simulink model "Hexa_CAD_ANSFT_Sim"  (R2024b)
settings: Solver=ode4  StartTime=0.0  StopTime=8  FixedStep=0.01  RelTol=1e-3
model workspace (MAT data in the model file):
  hover_2m = [0 0 2 0 0 0 0 0 2 0 0 0 ... (36 elements, 6x6)]
  square = [0 0 2.5 0 0 0 0 0 2.5 0 0 0 ... (36 elements, 6x6)]
  tf : Simulink.Parameter (value not decoded)
  tray0 = [0 0 0 0 0 0 0.2 0.15 2 0 0 0 ... (36 elements, 6x6)]
  tray1 = [0 0 0 0 0 0 0 0 5 0 0 0 ... (36 elements, 6x6)]
  tray2 = [0 0 0 0 0 0 2 0 5 0 0 0 ... (36 elements, 6x6)]
  tray3 = [0 0 0 0 0 0 2 0 5 0 0 0 ... (36 elements, 6x6)]
  tray4 = [0 0 0 0 0 0 2 0 5 0.15 0 0 ... (36 elements, 6x6)]
  tray5 = [0 0 0 0 0 0 0 0 5 0.15 0 0 ... (36 elements, 6x6)]
  tray_yaw = [0 0 0 0 0 0 0 0 5 0 0 0 ... (36 elements, 6x6)]
undefined symbols (not defined in the file or in its folder): F, Light, MIL, smiData, X, Y, Z
libraries: sm_lib x238, nesl_utility x29, dspobslib x7, simulink x3, sharedtransform x2, robotcorelib x1, aerolibwind2 x1
(part 2 of 6)

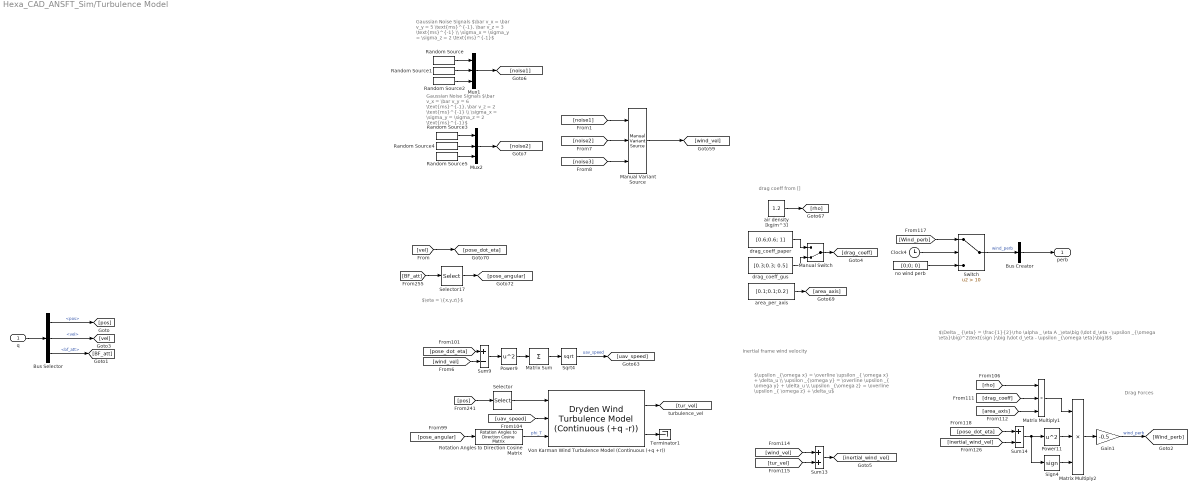
== system Hexa_CAD_ANSFT_Sim/Turbulence Model ==
  note: $\Delta _ {\eta} = \frac{1}{2}\rho \alpha _ \eta A _\eta\big (\dot d_\eta - \upsilon _{\omega \eta}\big)^2\text{sign }\big (\dot d_\eta - \upsilon _{\omega \eta}\big)$$
  note: $\upsilon _{\omega x} = \overline \upsilon _{ \omega x} + \delta_u \\ \upsilon _{\omega y} = \overline \upsilon _{ \omega y} + \delta_u \\ \upsilon _{\omega z} = \overline \upsilon _{ \omega z} + \delta_u$
  note: drag coeff from []
  note: Drag Forces
  note: Inertial frame wind velocity
  note: $\eta = \{x,y,z\}$
  note: Gaussian Noise Signals
      | $\bar v_x = \bar v_y = 6 \text{ms}^{-1}, \bar v_z = 2 \text{ms}^{-1} \\ \sigma_x = \sigma_y = \sigma_z = 2 \text{ms}^{-1}$
  note: Gaussian Noise Signals
      | $\bar v_x = \bar v_y = 5 \text{ms}^{-1}, \bar v_z = 3 \text{ms}^{-1} \\ \sigma_x = \sigma_y = \sigma_z = 2 \text{ms}^{-1}$
  q : Inport
  Bus Creator : BusCreator  Inputs=1
  Bus Selector : BusSelector  OutputSignals=pos,vel,bf_att
  Clock4 : Clock
  Gain1 : Gain  Gain=-0.5
  Manual Variant Source : simulink/Signal Routing/Manual Variant Source  NumChoices=3  LabelModeActiveChoice=V_1
  Manual Switch : ManualSwitch  CurrentSetting=0
  Matrix Sum : Sum  Inputs=+
  Matrix Multiply1 : Product  Inputs=3
  Matrix Multiply2 : Product  Inputs=3
  Mux1 : Mux  Inputs=3
  Mux2 : Mux  Inputs=3
  Power11 : Math  Operator=square
  Power9 : Math  Operator=square
  Random Source : dspobslib/Random Source  SrcType=Gaussian  NormMethod=Ziggurat  CltLength=12  MinVal=0  MaxVal=1  MeanVal=5  VarVal=2  RepMode=Not repeatable  rawSeed=1  IsInherit=off  SampMode=Discrete  SampTime=1  SampFrame=1  DataType=Double  OutComplex=Real  OutputFrames=off
  Random Source1 : dspobslib/Random Source  SrcType=Gaussian  NormMethod=Ziggurat  CltLength=12  MinVal=0  MaxVal=1  MeanVal=5  VarVal=2  RepMode=Not repeatable  rawSeed=1  IsInherit=off  SampMode=Discrete  SampTime=1  SampFrame=1  DataType=Double  OutComplex=Real  OutputFrames=off
  Random Source2 : dspobslib/Random Source  SrcType=Gaussian  NormMethod=Ziggurat  CltLength=12  MinVal=0  MaxVal=1  MeanVal=3  VarVal=2  RepMode=Not repeatable  rawSeed=1  IsInherit=off  SampMode=Discrete  SampTime=1  SampFrame=1  DataType=Double  OutComplex=Real  OutputFrames=off
  Random Source3 : dspobslib/Random Source  SrcType=Gaussian  NormMethod=Ziggurat  CltLength=12  MinVal=0  MaxVal=1  MeanVal=6  VarVal=2  RepMode=Not repeatable  rawSeed=1  IsInherit=off  SampMode=Discrete  SampTime=1  SampFrame=1  DataType=Double  OutComplex=Real  OutputFrames=off
  Random Source4 : dspobslib/Random Source  SrcType=Gaussian  NormMethod=Ziggurat  CltLength=12  MinVal=0  MaxVal=1  MeanVal=6  VarVal=2  RepMode=Not repeatable  rawSeed=1  IsInherit=off  SampMode=Discrete  SampTime=1  SampFrame=1  DataType=Double  OutComplex=Real  OutputFrames=off
  Random Source5 : dspobslib/Random Source  SrcType=Gaussian  NormMethod=Ziggurat  CltLength=12  MinVal=0  MaxVal=1  MeanVal=2  VarVal=2  RepMode=Not repeatable  rawSeed=1  IsInherit=off  SampMode=Discrete  SampTime=1  SampFrame=1  DataType=Double  OutComplex=Real  OutputFrames=off
  Rotation Angles to Direction Cosine Matrix : sharedtransform/Rotation Angles to Direction Cosine Matrix  rotationOrder=XYZ  aMode=aMode
  Selector : Selector  InputPortWidth=3  IndexOptions=Index vector (dialog)  Indices=[3]  OutputSizes=1
  Selector17 : Selector  InputPortWidth=3  IndexOptions=Index vector (dialog)  Indices=[3 2 1]  OutputSizes=1
  Sign4 : Signum
  Sqrt4 : Sqrt
  Sum13 : Sum
  Sum14 : Sum  Inputs=+-
  Sum9 : Sum  Inputs=+-
  Switch : Switch  Criteria=u2 > Threshold  Threshold=10  SaturateOnIntegerOverflow=off  InputSameDT=off
  Terminator1 : Terminator
  Von Karman Wind Turbulence Model (Continuous (+q +r)) : aerolibwind2/Dryden Wind Turbulence Model  (Continuous (+q -r))  units=Metric (MKS)  spec=MIL-F-8785C  model=Continuous Von Karman (+q -r)  W20=15  Wdeg=0  TurbProb=10^-2 - Light  L_high=762  Wingspan=10  ts=0.1  Seed=[23341 23342 23343 23344]  T_on=on
      settings: LibrarySourceBlock=|
      | aerolibwind2/Von Karman Wind Turbulence Model
      | (Continuous (+q +r))
  air density [kg/m^3] : Constant  Value=1.2
  area_per_axis : Constant  Value=[0.1;0.1;0.2]
  drag_coeff_gus : Constant  Value=[0.3;0.3; 0.5]
  drag_coeff_paper : Constant  Value=[0.6;0.6; 1]
  no wind perb : Constant  Value=[0;0; 0]
  perb : Outport
  wires:
  [rho] -> Matrix Multiply1/1
  [drag_coeff] -> Matrix Multiply1/2
  Von Karman Wind Turbulence Model (Continuous (+q +r))/2 -> Terminator1/1
  area_per_axis/1 -> [area_axis]
  [pose_dot_eta] -> Sum14/1
  Von Karman Wind Turbulence Model (Continuous (+q +r))/1 -> [tur_vel]
  [wind_vel] -> Sum9/2
  Selector17/1 -> [pose_angular]
  Matrix Multiply1/1 -> Matrix Multiply2/1
  Sign4/1 -> Matrix Multiply2/3
  [uav_speed] -> Von Karman Wind Turbulence Model (Continuous (+q +r))/2
  Power9/1 -> Matrix Sum/1
  Sqrt4/1 -> [uav_speed]  "uav_speed"
  Gain1/1 -> [Wind_perb]  "wind_perb"
  Sum9/1 -> Power9/1
  air density [kg/m^3]/1 -> [rho]
  Clock4/1 -> Switch/2
  [pose_dot_eta] -> Sum9/1
  Rotation Angles to Direction Cosine Matrix/1 -> Von Karman Wind Turbulence Model (Continuous (+q +r))/3  "phi_T"
  [tur_vel] -> Sum13/2
  Sum14/1 -> Sign4/1, Power11/1
  no wind perb/1 -> Switch/3
  drag_coeff_gus/1 -> Manual Switch/2
  Switch/1 -> Bus Creator/1  "wind_perb"
  [area_axis] -> Matrix Multiply1/3
  Manual Switch/1 -> [drag_coeff]
  Selector/1 -> Von Karman Wind Turbulence Model (Continuous (+q +r))/1
  [pose_angular] -> Rotation Angles to Direction Cosine Matrix/1
  [inertial_wind_vel] -> Sum14/2
  Matrix Multiply2/1 -> Gain1/1
  drag_coeff_paper/1 -> Manual Switch/1
  Power11/1 -> Matrix Multiply2/2
  Matrix Sum/1 -> Sqrt4/1
  Sum13/1 -> [inertial_wind_vel]
  [Wind_perb] -> Switch/1
  [wind_vel] -> Sum13/1
  Bus Creator/1 -> perb/1
  [BF_att] -> Selector17/1
  [pos] -> Selector/1
  q/1 -> Bus Selector/1
  Bus Selector/1 -> [pos]  "<pos>"
  Bus Selector/3 -> [BF_att]  "<bf_att>"
  Bus Selector/2 -> [vel]  "<vel>"
  [vel] -> [pose_dot_eta]
  Mux2/1 -> [noise2]
  Random Source5/1 -> Mux2/3
  Random Source/1 -> Mux1/1
  Mux1/1 -> [noise1]
  Random Source2/1 -> Mux1/3
  Random Source4/1 -> Mux2/2
  Random Source3/1 -> Mux2/1
  [noise2] -> Manual Variant Source/2
  Manual Variant Source/1 -> [wind_vel]
  Random Source1/1 -> Mux1/2
  [noise1] -> Manual Variant Source/1
  [noise3] -> Manual Variant Source/3

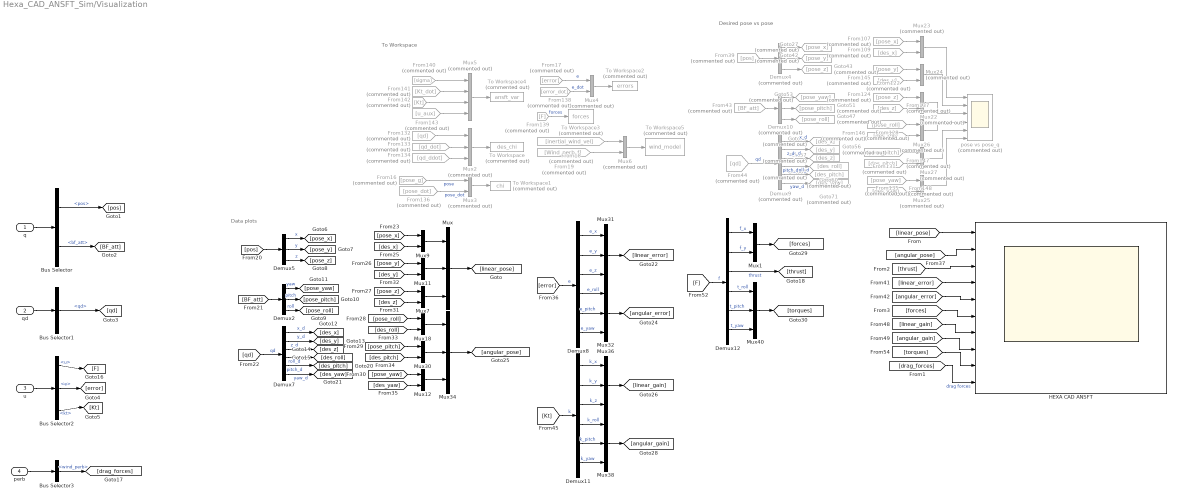
== system Hexa_CAD_ANSFT_Sim/Visualization ==
  note: Desired pose vs pose
  note: Data plots
  note: To Workspace
  q : Inport
  qd : Inport  Port=2
  u : Inport  Port=3
  perb : Inport  Port=4
  Bus Selector : BusSelector  OutputSignals=pos,bf_att
  Bus Selector1 : BusSelector  OutputSignals=qd
  Bus Selector2 : BusSelector  OutputSignals=u,e,kt
  Bus Selector3 : BusSelector  OutputSignals=wind_perb
  Demux10 : Demux  Commented=on  Outputs=3
  Demux{7..8,11..12} (4 alike) : Demux  Outputs=6
  Demux2 : Demux  Outputs=3
  Demux4 : Demux  Commented=on  Outputs=3
  Demux5 : Demux  Outputs=3
  Demux9 : Demux  Commented=on  Outputs=6
  From107 : From  Commented=on  GotoTag=pose_x
  From109 : From  Commented=on  GotoTag=des_x
  From122 : From  Commented=on  GotoTag=pose_y
  From124 : From  Commented=on  GotoTag=pose_z
  From128 : From  Commented=on  GotoTag=pose_roll
  From131 : From  Commented=on  GotoTag=pose_pitch
  From132 : From  Commented=on  GotoTag=qd
  From133 : From  Commented=on  GotoTag=qd_dot
  From134 : From  Commented=on  GotoTag=qd_ddot
  From135 : From  Commented=on  GotoTag=pose_yaw
  From136 : From  Commented=on  GotoTag=pose_dot
  From137 : From  Commented=on  GotoTag=des_z
  From138 : From  Commented=on  GotoTag=error_dot
  From139 : From  Commented=on  GotoTag=F
  From140 : From  Commented=on  GotoTag=sigma
  From141 : From  Commented=on  GotoTag=Kt_dot
  From142 : From  Commented=on  GotoTag=Kt
  From143 : From  Commented=on  GotoTag=u_aux
  From145 : From  Commented=on  GotoTag=des_y
  From146 : From  Commented=on  GotoTag=des_roll
  From147 : From  Commented=on  GotoTag=des_pitch
  From148 : From  Commented=on  GotoTag=des_yaw
  From16 : From  Commented=on  GotoTag=pose_g
  From17 : From  Commented=on  GotoTag=error
  From18 : From  Commented=on  GotoTag=inertial_wind_vel
  From19 : From  Commented=on  GotoTag=Wind_perb_f  TagVisibility=global
  From39 : From  Commented=on  GotoTag=pos
  From43 : From  Commented=on  GotoTag=BF_att
  From44 : From  Commented=on  GotoTag=qd
  Goto27 : Goto  Commented=on  GotoTag=pose_x
  Goto42 : Goto  Commented=on  GotoTag=pose_y
  Goto43 : Goto  Commented=on  GotoTag=pose_z
  Goto47 : Goto  Commented=on  GotoTag=pose_roll
  Goto51 : Goto  Commented=on  GotoTag=pose_pitch
  Goto53 : Goto  Commented=on  GotoTag=pose_yaw
  Goto55 : Goto  Commented=on  GotoTag=des_x
  Goto56 : Goto  Commented=on  GotoTag=des_y
  Goto57 : Goto  Commented=on  GotoTag=des_z
  Goto60 : Goto  Commented=on  GotoTag=des_roll
  Goto68 : Goto  Commented=on  GotoTag=des_pitch
  Goto71 : Goto  Commented=on  GotoTag=des_yaw
  HEXA CAD ANSFT : Scope  NumInputPorts=10
  Mux{,31..32,34,36,38,40} (7 alike) : Mux  Inputs=3
  Mux{1,7,9,11..12,18,30} (7 alike) : Mux  Inputs=2
  Mux2 : Mux  Commented=on  Inputs=3
  Mux{3..4,6,22..27} (9 alike) : Mux  Commented=on  Inputs=2
  Mux5 : Mux  Commented=on
  To Workspace : ToWorkspace  Commented=on  VariableName=des_chi  SaveFormat=Structure With Time  SampleTime=-1
  To Workspace1 : ToWorkspace  Commented=on  VariableName=chi  SaveFormat=Structure With Time  SampleTime=-1
  To Workspace2 : ToWorkspace  Commented=on  VariableName=errors  SaveFormat=Structure With Time  SampleTime=-1
  To Workspace3 : ToWorkspace  Commented=on  VariableName=forces  SaveFormat=Structure With Time  SampleTime=-1
  To Workspace4 : ToWorkspace  Commented=on  VariableName=ansft_var  SaveFormat=Structure With Time  SampleTime=-1
  To Workspace5 : ToWorkspace  Commented=on  VariableName=wind_model  SaveFormat=Structure With Time  SampleTime=-1
  pose vs pose_q : Scope  Commented=on  NumInputPorts=6
  wires:
  Mux/1 -> [linear_pose]
  Mux6/1 -> To Workspace5/1
  Mux9/1 -> Mux/1
  From128/1 -> Mux26/1
  Demux4/1 -> Goto27/1
  Demux7/5 -> [des_pitch]  "pitch_d"
  From135/1 -> Mux25/1
  [linear_error] -> HEXA CAD ANSFT/4
  [angular_error] -> HEXA CAD ANSFT/5
  From132/1 -> Mux2/1
  Mux11/1 -> Mux/2
  Demux11/2 -> Mux36/2  "k_y"
  Demux4/3 -> Goto43/1
  Demux5/1 -> [pose_x]  "x"
  Demux10/1 -> Goto53/1
  Demux12/6 -> Mux40/3  "t_yaw"
  Demux12/4 -> Mux40/1  "t_roll"
  Mux40/1 -> [torques]
  Mux1/1 -> [forces]
  Demux10/3 -> Goto47/1
  Mux3/1 -> To Workspace1/1
  Demux5/3 -> [pose_z]  "z"
  Demux11/1 -> Mux36/1  "k_x"
  Demux8/6 -> Mux32/3  "e_yaw"
  From148/1 -> Mux25/2
  Demux11/4 -> Mux38/1  "k_roll"
  Demux9/6 -> Goto71/1  "yaw_d"
  [BF_att] -> Demux2/1
  Mux31/1 -> [linear_error]
  Mux23/1 -> pose vs pose_q/1
  Demux9/2 -> Goto56/1  "y_d"
  Demux7/2 -> [des_y]  "y_d"
  Demux5/2 -> [pose_y]  "y"
  From16/1 -> Mux3/1  "pose"
  [pose_pitch] -> Mux30/1
  [pose_y] -> Mux11/1
  Demux8/3 -> Mux31/3  "e_z"
  From44/1 -> Demux9/1  "qd"
  Demux7/3 -> [des_z]  "z_d"
  Demux12/2 -> Mux1/2  "f_y"
  [angular_gain] -> HEXA CAD ANSFT/8
  [error] -> Demux8/1  "e"
  From133/1 -> Mux2/2
  [des_pitch] -> Mux30/2
  [F] -> Demux12/1  "f"
  Mux5/1 -> To Workspace4/1
  [linear_gain] -> HEXA CAD ANSFT/7
  Mux2/1 -> To Workspace/1
  [des_roll] -> Mux18/2
  From43/1 -> Demux10/1
  Mux22/1 -> pose vs pose_q/3
  Mux26/1 -> pose vs pose_q/4
  Mux24/1 -> pose vs pose_q/2
  Demux12/1 -> Mux1/1  "f_x"
  From109/1 -> Mux23/2
  Demux7/4 -> [des_roll]  "roll_d"
  Demux9/4 -> Goto60/1  "roll_d"
  Demux12/3 -> [thrust]  "thrust"
  From122/1 -> Mux24/1
  Mux36/1 -> [linear_gain]
  [des_yaw] -> Mux12/2
  Demux11/6 -> Mux38/3  "k_yaw"
  From139/1 -> To Workspace3/1  "forces"
  [angular_pose] -> HEXA CAD ANSFT/2
  Demux9/3 -> Goto57/1  "z_d"
  Demux8/1 -> Mux31/1  "e_x"
  Demux2/3 -> [pose_roll]  "roll"
  From124/1 -> Mux22/1
  Demux7/1 -> [des_x]  "x_d"
  From138/1 -> Mux4/2  "e_dot"
  [pose_yaw] -> Mux12/1
  Demux2/1 -> [pose_yaw]  "yaw"
  Demux2/2 -> [pose_pitch]  "pitch"
  From39/1 -> Demux4/1
  From137/1 -> Mux22/2
  Mux12/1 -> Mux34/3
  From131/1 -> Mux27/1
  Demux12/5 -> Mux40/2  "t_pitch"
  [des_x] -> Mux9/2
  Demux8/4 -> Mux32/1  "e_roll"
  [linear_pose] -> HEXA CAD ANSFT/1
  Demux9/1 -> Goto55/1  "x_d"
  [pos] -> Demux5/1
  From18/1 -> Mux6/1
  From141/1 -> Mux5/2
  Mux7/1 -> Mux/3
  From145/1 -> Mux24/2
  Demux9/5 -> Goto68/1  "pitch_d"
  From17/1 -> Mux4/1  "e"
  Demux8/5 -> Mux32/2  "e_pitch"
  Mux34/1 -> [angular_pose]
  [pose_x] -> Mux9/1
  Demux10/2 -> Goto51/1
  [pose_roll] -> Mux18/1
  [pose_z] -> Mux7/1
  Mux30/1 -> Mux34/2
  [des_y] -> Mux11/2
  Demux11/3 -> Mux36/3  "k_z"
  Demux7/6 -> [des_yaw]  "yaw_d"
  Mux4/1 -> To Workspace2/1
  From19/1 -> Mux6/2
  From134/1 -> Mux2/3
  Mux38/1 -> [angular_gain]
  Mux18/1 -> Mux34/1
  Demux11/5 -> Mux38/2  "k_pitch"
  Demux4/2 -> Goto42/1
  [Kt] -> Demux11/1  "k"
  Mux32/1 -> [angular_error]
  [qd] -> Demux7/1  "qd"
  Demux8/2 -> Mux31/2  "e_y"
  From143/1 -> Mux5/4
  From146/1 -> Mux26/2
  Mux27/1 -> pose vs pose_q/5
  [des_z] -> Mux7/2
  From147/1 -> Mux27/2
  From142/1 -> Mux5/3
  From140/1 -> Mux5/1
  From136/1 -> Mux3/2  "pose_dot"
  From107/1 -> Mux23/1
  Mux25/1 -> pose vs pose_q/6
  q/1 -> Bus Selector/1
  Bus Selector/1 -> [pos]  "<pos>"
  Bus Selector/2 -> [BF_att]  "<bf_att>"
  qd/1 -> Bus Selector1/1
  Bus Selector1/1 -> [qd]  "<qd>"
  u/1 -> Bus Selector2/1
  Bus Selector2/1 -> [F]  "<u>"
  Bus Selector2/2 -> [error]  "<e>"
  Bus Selector2/3 -> [Kt]  "<kt>"
  perb/1 -> Bus Selector3/1
  Bus Selector3/1 -> [drag_forces]  "<wind_perb>"
  [thrust] -> HEXA CAD ANSFT/3
  [forces] -> HEXA CAD ANSFT/6
  [torques] -> HEXA CAD ANSFT/9
  [drag_forces] -> HEXA CAD ANSFT/10  "drag forces"
